simulink model "simulation"  (R2021b)
settings: Solver=FixedStepAuto  StartTime=0.0  StopTime=T  RelTol=1e-3  EnableMultiTasking=on
undefined symbols (not defined in the file or in its folder): constgain, discrete_0, h, Humusoft, K, MF634
libraries: sldrtlib x2, eeLuenbergerObserver x1, simulink x1
settings Model: Creator=rbabuska  LastModifiedBy=wterhaar
settings SolverCC: AlgebraicLoopSolver=TrustRegion  AutoInsertRateTranBlk=on
settings DataIOCC: LimitDataPoints=on  SaveFormat=Array  SignalLoggingSaveFormat=ModelDataLogs  SaveOutput=off  SaveTime=off  ReturnWorkspaceOutputs=off
settings OptimizationCC: DefaultParameterBehavior=Inlined  InlineInvariantSignals=on  EnhancedBackFolding=on  PassReuseOutputArgsAs=Individual arguments  ExpressionDepthLimit=2147483647  StateBitsets=on  DataBitsets=on  ZeroExternalMemoryAtStartup=off  ZeroInternalMemoryAtStartup=off  NoFixptDivByZeroProtection=on  LifeSpan=1  OptimizeBlockOrder=speed  DifferentSizesBufferReuse=on  EfficientTunableParamExpr=on
settings DebuggingCC: UnderspecifiedInitializationDetection=Classic  MergeDetectMultiDrivingBlocksExec=none  ParameterTunabilityLossMsg=error  FcnCallInpInsideContextMsg=warning  StateNameClashWarn=warning  SFUnexpectedBacktrackingDiag=warning  SFNoUnconditionalDefaultTransitionDiag=warning  SFExecutionAtInitializationDiag=none  SFMachineParentedDataDiag=warning  ArithmeticOperatorsInVariantConditions=warning
settings HardwareCC: ProdBitPerPointer=32  ProdBitPerSizeT=32  ProdBitPerPtrDiffT=32  ProdLargestAtomicFloat=None  ProdIntDivRoundTo=Floor  ProdWordSize=32  ProdHWDeviceType=Generic->Custom
settings ModelReferenceCC: PropagateSignalLabelsOutOfModel=off
settings SFSimCC: SimUseLocalCustomCode=off  MATLABDynamicMemAlloc=off  CustomCodeUndefinedFunction=UseInterfaceOnly
settings RTWCC: Description=Embedded Coder  SystemTargetFile=ert.tlc  TLCOptions=-p0  GenCodeOnly=on  TemplateMakefile=ert_default_tmf  GenerateReport=on  RTWVerbose=off  RTWUseLocalCustomCode=off  IncludeHyperlinkInReport=on  LaunchReport=on
settings CodeAppCC: ForceParamTrailComments=on  IgnoreCustomStorageClasses=off  OperatorAnnotations=on  SimulinkDataObjDesc=on  SFDataObjDesc=on  CustomSymbolStrGlobalVar=rt$N$M  CustomSymbolStrType=$N$M  CustomSymbolStrFcn=$N$M$F  CustomSymbolStrMacro=$N$M  InsertBlockDesc=on
settings ERTTargetCC: CodeReplacementLibrary=ISO_C  GenerateSampleERTMain=on  IncludeMdlTerminateFcn=off  SuppressErrorStatus=on  SupportAbsoluteTime=off  PurelyIntegerCode=on  SupportNonFinite=off  SupportComplex=off  InlinedParameterPlacement=NonHierarchical  RootIOFormat=Structure reference  ERTCustomFileTemplate=example_file_process.tlc
settings ConfigComp: CovMetricSettings=dw  CovSaveCumulativeToWorkspaceVar=on  CovSaveSingleToWorkspaceVar=on  CovExternalEMLEnable=off  CovSFcnEnable=off

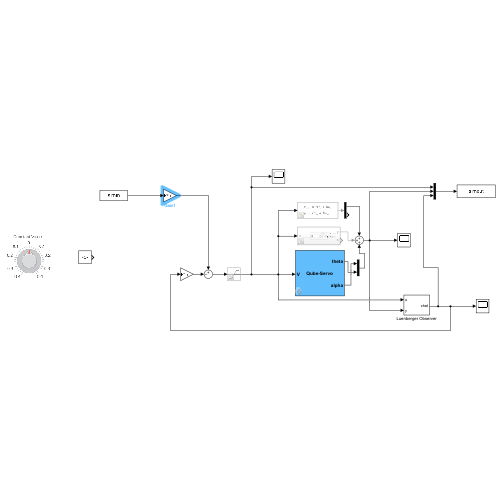
[thumbnail: Simulink's stored preview of the top-level diagram]
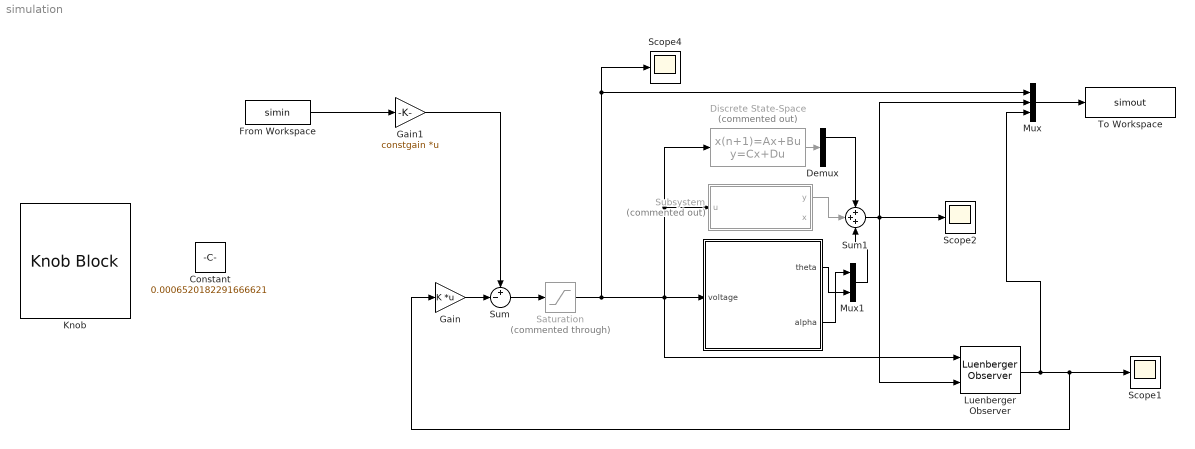
== system simulation ==
  " " : Subsystem  LoadFcn=hwinit  InitFcn=hwinit  mask{h=h}
      mask prompts: h "Sampling period [s]"
      mask Display:
      | disp('Qube-Servo')
      | port_label('output',1,'theta')
      | port_label('output',2,'alpha')
      | port_label('input',1,'V')
  Constant : Constant  Value=0.0006520182291666621
  Demux : Demux  Outputs=[2;4]
  Discrete State-Space : DiscreteStateSpace  Commented=on  A=discrete_0.A  B=discrete_0.B  C=[discrete_0.C;eye(4)]  D=[discrete_0.D;zeros(4,1)]  InitialCondition=[0;0;0;0]  SampleTime=h
  From Workspace : FromWorkspace  VariableName=simin  SampleTime=h  OutputAfterFinalValue=Holding final value
  Gain : Gain  Gain=K  Multiplication=Matrix(K*u)
  Gain1 : Gain  Gain=constgain  Multiplication=Matrix(K*u)
  Knob : KnobBlock  ScaleMin=-0.4  ScaleMax=0.4
  Luenberger Observer : eeLuenbergerObserver/Luenberger Observer  StateSpaceType=Discrete-time  Ad=discrete_0.A  Bd=discrete_0.B  Cd=discrete_0.C  Dd=discrete_0.D  A=1  B=1  C=1  D=1  ObserverDesign=Observer gain  Ld=disc  DesiredEigenvalues=pDisc  x0=[0;0;0;0]  Tsd=0.1  Ts=h
      settings: SourceProductBaseCode=PS
  Mux : Mux  Inputs=3
  Mux1 : Mux  Inputs=2
  Saturation : Saturate  Commented=through  UpperLimit=0.2  LowerLimit=-0.2
  Scope1 : Scope
  Scope2 : Scope
  Scope4 : Scope
  Subsystem : Subsystem  Commented=on
  Sum : Sum  Inputs=+-|
  Sum1 : Sum  Inputs=+++
  To Workspace : ToWorkspace  VariableName=simout  SaveFormat=Timeseries  SampleTime=-1
  wires:
  Mux/1 -> To Workspace/1
  Luenberger Observer/1 -> Mux/3, Gain/1, Scope1/1
  Discrete State-Space/1 -> Demux/1
  Sum1/1 -> Luenberger Observer/2, Mux/2, Scope2/1
  Saturation/1 -> " "/1(voltage), Luenberger Observer/1, Subsystem/1(u), Discrete State-Space/1, Scope4/1, Mux/1
  " "/2(alpha) -> Mux1/1
  " "/1(theta) -> Mux1/2
  Mux1/1 -> Sum1/3
  Subsystem/1(y) -> Sum1/2
  Demux/1 -> Sum1/1
  From Workspace/1 -> Gain1/1
  Sum/1 -> Saturation/1
  Gain/1 -> Sum/2
  Gain1/1 -> Sum/1

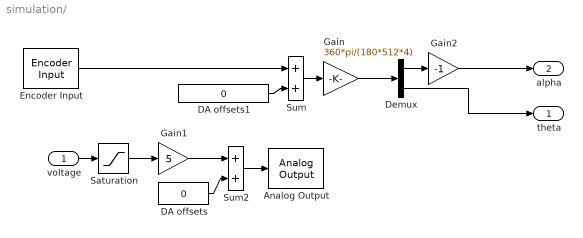
== system simulation/  ==
  voltage : Inport
  Analog Output : sldrtlib/Analog Output  SampleTime=h  MaxMissedTicks=100  ShowMissedTicks=off  YieldWhenWaiting=off  DrvName=Humusoft/MF634  DrvAddress=4294967295  DrvOptions=0  Channels=[1]  RangeMode=2  VoltRange=1  InitialValue=0  FinalValue=0
      settings: AttributesFormatString=Humusoft\nMF634 [auto]
  DA offsets : Constant  Value=0
  DA offsets1 : Constant  Value=0  SampleTime=h
  Demux : Demux  Outputs=2
  Encoder Input : sldrtlib/Encoder Input  SampleTime=h  MaxMissedTicks=100  ShowMissedTicks=off  YieldWhenWaiting=off  DrvName=Humusoft/MF634  DrvAddress=4294967295  DrvOptions=0  Channels=[1,2]  QuadMode=3  IndexPulse=1  InputFilter=Inf  DataType=1
      settings: AttributesFormatString=Humusoft\nMF634 [auto]
  Gain : Gain  Gain=360*pi/(180*512*4)  SaturateOnIntegerOverflow=on  OutDataTypeStr=Inherit: Same as input  ParamDataTypeStr=Inherit: Same as input
  Gain1 : Gain  Gain=5  SaturateOnIntegerOverflow=on  OutDataTypeStr=Inherit: Same as input  ParamDataTypeStr=Inherit: Same as input
  Gain2 : Gain  Gain=-1  SaturateOnIntegerOverflow=on  OutDataTypeStr=Inherit: Same as input  ParamDataTypeStr=Inherit: Same as input
  Saturation : Saturate  UpperLimit=1  LowerLimit=-1
  Sum : Sum  InputSameDT=on  SaturateOnIntegerOverflow=on  OutDataTypeStr=Inherit: Same as first input
  Sum2 : Sum  InputSameDT=on  SaturateOnIntegerOverflow=on  OutDataTypeStr=Inherit: Same as first input
  theta : Outport  Tag=Cable length
  alpha : Outport  Tag=Cable length  Port=2
  wires:
  Sum/1 -> Gain/1
  DA offsets1/1 -> Sum/2
  Gain1/1 -> Sum2/1
  Sum2/1 -> Analog Output/1
  DA offsets/1 -> Sum2/2
  voltage/1 -> Saturation/1
  Encoder Input/1 -> Sum/1
  Saturation/1 -> Gain1/1
  Demux/1 -> Gain2/1
  Gain/1 -> Demux/1
  Gain2/1 -> alpha/1
  Demux/2 -> theta/1

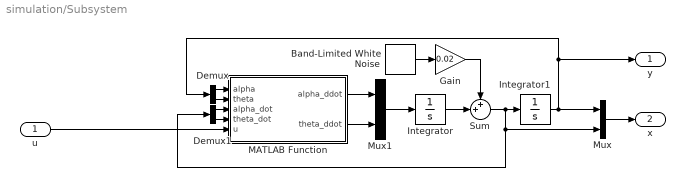
== system simulation/Subsystem ==
  u : Inport
  Band-Limited White Noise : simulink/Sources/Band-Limited White Noise  Cov=[0.02]  Ts=0.1  seed=[23341]
  Demux : Demux  Outputs=2
  Demux1 : Demux  Outputs=2
  Gain : Gain  Gain=0.02
  Integrator : Integrator
  Integrator1 : Integrator
  MATLAB Function : MATLAB Function  TreatAsAtomicUnit=on
  Mux : Mux  Inputs=2
  Mux1 : Mux  Inputs=2
  Sum : Sum  Inputs=++|
  y : Outport  PortDimensions=2
  x : Outport  Port=2  PortDimensions=4
  wires:
  Integrator/1 -> Sum/2
  Sum/1 -> Mux/2, Demux1/1, Integrator1/1
  MATLAB Function/2(theta_ddot) -> Mux1/2
  MATLAB Function/1(alpha_ddot) -> Mux1/1
  Demux/2 -> MATLAB Function/2(theta)
  Demux/1 -> MATLAB Function/1(alpha)
  Integrator1/1 -> Demux/1, y/1, Mux/1
  Mux1/1 -> Integrator/1
  Demux1/2 -> MATLAB Function/4(theta_dot)
  Demux1/1 -> MATLAB Function/3(alpha_dot)
  u/1 -> MATLAB Function/5(u)
  Mux/1 -> x/1
  Band-Limited White Noise/1 -> Gain/1
  Gain/1 -> Sum/1

== matlab function simulation/Subsystem/MATLAB Function ==
  data: alpha input; theta input; alpha_dot input; theta_dot input; alpha_ddot output; u input; theta_ddot output
function [alpha_ddot,theta_ddot] = fcn(alpha,theta,alpha_dot,theta_dot,u)
alpha_ddot=((alpha_dot.*(-2.46872604672e-5)+u.*1.9980288e-3+theta_dot.^2.*sin(theta).*9.47552256e-7+cos(theta).*sin(theta).*4.5993298176e-4+theta_dot.*cos(theta).*8.22528e-7).*(-5.0./8.4e+1))./(cos(theta).^2.*5.992704e-8-1.4533632e-7);
theta_ddot=((theta_dot.*1.059744e-6+sin(theta).*5.9257705248e-4-alpha_dot.*cos(theta).*1.31151071232e-5+u.*cos(theta).*1.0614528e-3+theta_dot.^2.*cos(theta).*sin(theta).*5.03387136e-7).*(5.0./4.2e+1))./(cos(theta).^2.*5.992704e-8-1.4533632e-7);
